simulink library "monroe_library"  (R2012b)
settings: Solver=ode45  StartTime=0.0  StopTime=10.0  RelTol=1e-3
values from neighbouring files (symbols this model uses):
  input_bit_width = ', num2str(input_bit_width))    [fft_direct_draw.m]
undefined symbols (not defined in the file or in its folder): gcbh, xlBlockLoadCallback
libraries: xbsIndex_r4 x1880, monroe_library x159, casper_library x13, xps_library x1
(part 12 of 43)

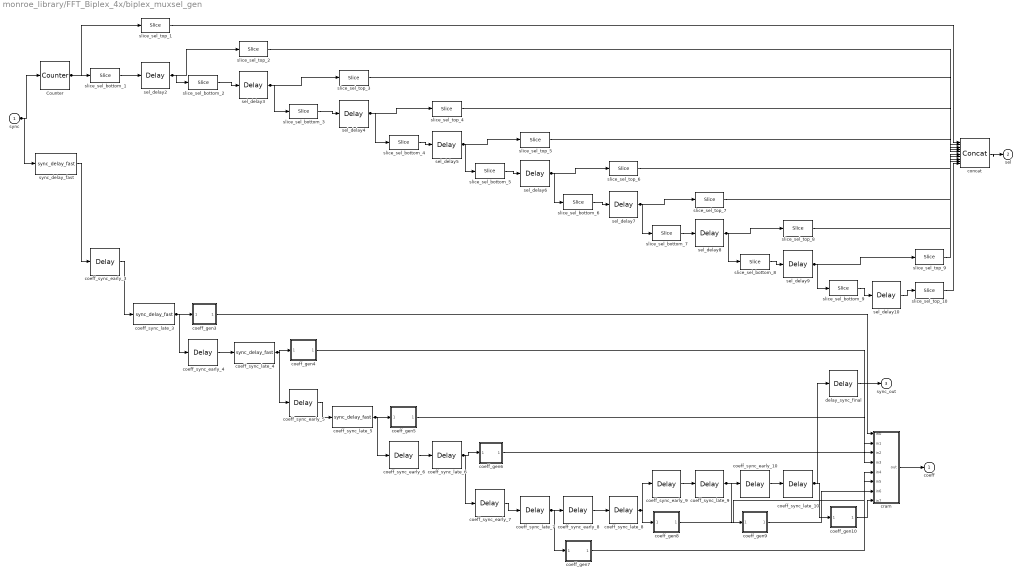
== system monroe_library/FFT_Biplex_4x/biplex_muxsel_gen ==
  sync : Inport
  Counter : xbsIndex_r4/Counter  cnt_type=Free Running  cnt_to=Inf  operation=Up  start_count=0  cnt_by_val=1  arith_type=Unsigned  n_bits=10  bin_pt=0  load_pin=off  rst=on  en=off  explicit_period=on  period=1  dbl_ovrd=off  use_behavioral_HDL=off  implementation=Fabric  block_type=counter
  coeff_gen10 : Subsystem
  coeff_gen3 : Subsystem
  coeff_gen4 : Subsystem
  coeff_gen5 : Subsystem
  coeff_gen6 : Subsystem
  coeff_gen7 : Subsystem
  coeff_gen8 : Subsystem
  coeff_gen9 : Subsystem
  coeff_sync_early_{4..10} (7 alike) : xbsIndex_r4/Delay  en=off  latency=6  dbl_ovrd=off  reg_retiming=off  block_type=delay
  coeff_sync_early_3 : xbsIndex_r4/Delay  en=off  latency=7  dbl_ovrd=off  reg_retiming=off  block_type=delay
  coeff_sync_late_10 : xbsIndex_r4/Delay  en=off  latency=1  dbl_ovrd=off  reg_retiming=off  block_type=delay
  coeff_sync_late_3 : monroe_library/sync_delay_fast  SystemSampleTime=-1  delay_len=128
  coeff_sync_late_4 : monroe_library/sync_delay_fast  SystemSampleTime=-1  delay_len=64
  coeff_sync_late_5 : monroe_library/sync_delay_fast  SystemSampleTime=-1  delay_len=32
  coeff_sync_late_6 : xbsIndex_r4/Delay  en=off  latency=16  dbl_ovrd=off  reg_retiming=off  block_type=delay
  coeff_sync_late_7 : xbsIndex_r4/Delay  en=off  latency=8  dbl_ovrd=off  reg_retiming=off  block_type=delay
  coeff_sync_late_8 : xbsIndex_r4/Delay  en=off  latency=4  dbl_ovrd=off  reg_retiming=off  block_type=delay
  coeff_sync_late_9 : xbsIndex_r4/Delay  en=off  latency=2  dbl_ovrd=off  reg_retiming=off  block_type=delay
  concat : xbsIndex_r4/Concat  num_inputs=10  dbl_ovrd=off  block_type=concat
  cram : Subsystem
  delay_sync_final : xbsIndex_r4/Delay  en=off  latency=6  dbl_ovrd=off  reg_retiming=off  block_type=delay
  sel_delay{4..10} (7 alike) : xbsIndex_r4/Delay  en=off  latency=6  dbl_ovrd=off  reg_retiming=off  block_type=delay
  sel_delay2 : xbsIndex_r4/Delay  en=off  latency=2  dbl_ovrd=off  reg_retiming=off  block_type=delay
  sel_delay3 : xbsIndex_r4/Delay  en=off  latency=5  dbl_ovrd=off  reg_retiming=off  block_type=delay
  slice_sel_bottom_1 : xbsIndex_r4/Slice  nbits=9  boolean_output=off  mode=Lower Bit Location + Width  bit1=0  base1=LSB of Input  bit0=0  base0=LSB of Input  dbl_ovrd=off  block_type=slice
  slice_sel_bottom_2 : xbsIndex_r4/Slice  nbits=8  boolean_output=off  mode=Lower Bit Location + Width  bit1=0  base1=LSB of Input  bit0=0  base0=LSB of Input  dbl_ovrd=off  block_type=slice
  slice_sel_bottom_3 : xbsIndex_r4/Slice  nbits=7  boolean_output=off  mode=Lower Bit Location + Width  bit1=0  base1=LSB of Input  bit0=0  base0=LSB of Input  dbl_ovrd=off  block_type=slice
  slice_sel_bottom_4 : xbsIndex_r4/Slice  nbits=6  boolean_output=off  mode=Lower Bit Location + Width  bit1=0  base1=LSB of Input  bit0=0  base0=LSB of Input  dbl_ovrd=off  block_type=slice
  slice_sel_bottom_5 : xbsIndex_r4/Slice  nbits=5  boolean_output=off  mode=Lower Bit Location + Width  bit1=0  base1=LSB of Input  bit0=0  base0=LSB of Input  dbl_ovrd=off  block_type=slice
  slice_sel_bottom_6 : xbsIndex_r4/Slice  nbits=4  boolean_output=off  mode=Lower Bit Location + Width  bit1=0  base1=LSB of Input  bit0=0  base0=LSB of Input  dbl_ovrd=off  block_type=slice
  slice_sel_bottom_7 : xbsIndex_r4/Slice  nbits=3  boolean_output=off  mode=Lower Bit Location + Width  bit1=0  base1=LSB of Input  bit0=0  base0=LSB of Input  dbl_ovrd=off  block_type=slice
  slice_sel_bottom_8 : xbsIndex_r4/Slice  nbits=2  boolean_output=off  mode=Lower Bit Location + Width  bit1=0  base1=LSB of Input  bit0=0  base0=LSB of Input  dbl_ovrd=off  block_type=slice
  slice_sel_bottom_9 : xbsIndex_r4/Slice  nbits=1  boolean_output=off  mode=Lower Bit Location + Width  bit1=0  base1=LSB of Input  bit0=0  base0=LSB of Input  dbl_ovrd=off  block_type=slice
  slice_sel_top_{1..10} (10 alike) : xbsIndex_r4/Slice  nbits=1  boolean_output=on  mode=Upper Bit Location + Width  bit1=0  base1=MSB of Input  bit0=0  base0=MSB of Input  dbl_ovrd=off  block_type=slice
  sync_delay_fast : monroe_library/sync_delay_fast  SystemSampleTime=-1  delay_len=768
  coeff : Outport
  sel : Outport  Port=2
  sync_out : Outport  Port=3
  wires:
  sync/1 -> Counter/1, sync_delay_fast/1
  coeff_sync_late_3/1 -> coeff_sync_early_4/1, coeff_gen3/1(sync)
  coeff_sync_late_4/1 -> coeff_sync_early_5/1, coeff_gen4/1(sync)
  coeff_sync_late_5/1 -> coeff_sync_early_6/1, coeff_gen5/1(sync)
  coeff_sync_late_6/1 -> coeff_sync_early_7/1, coeff_gen6/1(sync)
  coeff_sync_late_7/1 -> coeff_sync_early_8/1, coeff_gen7/1(sync)
  coeff_sync_late_8/1 -> coeff_sync_early_9/1, coeff_gen8/1(sync)
  coeff_sync_late_9/1 -> coeff_sync_early_10/1, coeff_gen9/1(sync)
  coeff_sync_late_10/1 -> delay_sync_final/1, coeff_gen10/1(sync)
  Counter/1 -> slice_sel_bottom_1/1, slice_sel_top_1/1
  sel_delay2/1 -> slice_sel_bottom_2/1, slice_sel_top_2/1
  sel_delay3/1 -> slice_sel_bottom_3/1, slice_sel_top_3/1
  sel_delay4/1 -> slice_sel_bottom_4/1, slice_sel_top_4/1
  sel_delay5/1 -> slice_sel_bottom_5/1, slice_sel_top_5/1
  sel_delay6/1 -> slice_sel_bottom_6/1, slice_sel_top_6/1
  sel_delay7/1 -> slice_sel_bottom_7/1, slice_sel_top_7/1
  sel_delay8/1 -> slice_sel_bottom_8/1, slice_sel_top_8/1
  sel_delay9/1 -> slice_sel_bottom_9/1, slice_sel_top_9/1
  delay_sync_final/1 -> sync_out/1
  concat/1 -> sel/1
  slice_sel_top_10/1 -> concat/10
  slice_sel_top_9/1 -> concat/9
  slice_sel_top_8/1 -> concat/8
  slice_sel_top_7/1 -> concat/7
  slice_sel_top_6/1 -> concat/6
  slice_sel_top_5/1 -> concat/5
  slice_sel_top_4/1 -> concat/4
  slice_sel_top_3/1 -> concat/3
  slice_sel_top_2/1 -> concat/2
  slice_sel_top_1/1 -> concat/1
  sel_delay10/1 -> slice_sel_top_10/1
  slice_sel_bottom_9/1 -> sel_delay10/1
  slice_sel_bottom_8/1 -> sel_delay9/1
  slice_sel_bottom_7/1 -> sel_delay8/1
  slice_sel_bottom_6/1 -> sel_delay7/1
  slice_sel_bottom_5/1 -> sel_delay6/1
  slice_sel_bottom_4/1 -> sel_delay5/1
  slice_sel_bottom_3/1 -> sel_delay4/1
  slice_sel_bottom_2/1 -> sel_delay3/1
  slice_sel_bottom_1/1 -> sel_delay2/1
  cram/1(out) -> coeff/1
  coeff_gen10/1(coeff) -> cram/8(in7)
  coeff_gen9/1(coeff) -> cram/7(in6)
  coeff_gen8/1(coeff) -> cram/6(in5)
  coeff_gen7/1(coeff) -> cram/5(in4)
  coeff_gen6/1(coeff) -> cram/4(in3)
  coeff_gen5/1(coeff) -> cram/3(in2)
  coeff_gen4/1(coeff) -> cram/2(in1)
  coeff_gen3/1(coeff) -> cram/1(in0)
  coeff_sync_early_10/1 -> coeff_sync_late_10/1
  coeff_sync_early_9/1 -> coeff_sync_late_9/1
  coeff_sync_early_8/1 -> coeff_sync_late_8/1
  coeff_sync_early_7/1 -> coeff_sync_late_7/1
  coeff_sync_early_6/1 -> coeff_sync_late_6/1
  coeff_sync_early_5/1 -> coeff_sync_late_5/1
  coeff_sync_early_4/1 -> coeff_sync_late_4/1
  coeff_sync_early_3/1 -> coeff_sync_late_3/1
  sync_delay_fast/1 -> coeff_sync_early_3/1

== system monroe_library/FFT_Biplex_4x/cram0 ==
  in0 : Inport
  in1 : Inport  Port=2
  concat : xbsIndex_r4/Concat  num_inputs=2  dbl_ovrd=off  block_type=concat
  reinterpret_1 : xbsIndex_r4/Reinterpret  force_arith_type=on  arith_type=Unsigned  force_bin_pt=on  bin_pt=0  block_type=reinterpret
      settings: infoedit="Changes signal type without altering the binary representation.   You can changed the signal between signed and unsigned, and relocate the binary point.<br><br>Hardware notes: In hardware this block costs nothing.<br><br>Example:  Suppose the input is 6 bits wide, signed, with 2 fractional bits, and the output is forced to unsigned with 0 fractional bits.  Then an input of -2.0 (1110.00 in binary 2's complement) becomes an output of 56 (111000 in binary)."
  reinterpret_2 : xbsIndex_r4/Reinterpret  force_arith_type=on  arith_type=Unsigned  force_bin_pt=on  bin_pt=0  block_type=reinterpret
      settings: infoedit="Changes signal type without altering the binary representation.   You can changed the signal between signed and unsigned, and relocate the binary point.<br><br>Hardware notes: In hardware this block costs nothing.<br><br>Example:  Suppose the input is 6 bits wide, signed, with 2 fractional bits, and the output is forced to unsigned with 0 fractional bits.  Then an input of -2.0 (1110.00 in binary 2's complement) becomes an output of 56 (111000 in binary)."
  out : Outport
  wires:
  concat/1 -> out/1
  reinterpret_2/1 -> concat/2
  reinterpret_1/1 -> concat/1
  in1/1 -> reinterpret_2/1
  in0/1 -> reinterpret_1/1

== system monroe_library/FFT_Biplex_4x/cram1 ==
  in0 : Inport
  in1 : Inport  Port=2
  concat : xbsIndex_r4/Concat  num_inputs=2  dbl_ovrd=off  block_type=concat
  reinterpret_1 : xbsIndex_r4/Reinterpret  force_arith_type=on  arith_type=Unsigned  force_bin_pt=on  bin_pt=0  block_type=reinterpret
      settings: infoedit="Changes signal type without altering the binary representation.   You can changed the signal between signed and unsigned, and relocate the binary point.<br><br>Hardware notes: In hardware this block costs nothing.<br><br>Example:  Suppose the input is 6 bits wide, signed, with 2 fractional bits, and the output is forced to unsigned with 0 fractional bits.  Then an input of -2.0 (1110.00 in binary 2's complement) becomes an output of 56 (111000 in binary)."
  reinterpret_2 : xbsIndex_r4/Reinterpret  force_arith_type=on  arith_type=Unsigned  force_bin_pt=on  bin_pt=0  block_type=reinterpret
      settings: infoedit="Changes signal type without altering the binary representation.   You can changed the signal between signed and unsigned, and relocate the binary point.<br><br>Hardware notes: In hardware this block costs nothing.<br><br>Example:  Suppose the input is 6 bits wide, signed, with 2 fractional bits, and the output is forced to unsigned with 0 fractional bits.  Then an input of -2.0 (1110.00 in binary 2's complement) becomes an output of 56 (111000 in binary)."
  out : Outport
  wires:
  concat/1 -> out/1
  reinterpret_2/1 -> concat/2
  reinterpret_1/1 -> concat/1
  in1/1 -> reinterpret_2/1
  in0/1 -> reinterpret_1/1

== system monroe_library/FFT_Biplex_4x/stage_1 ==
  a : Inport
  b : Inport  Port=2
  sync : Inport  Port=3
  mux_sel : Inport  Port=4
  Mux : xbsIndex_r4/Mux  inputs=2  en=off  latency=0  precision=Full  arith_type="Signed  (2's comp)"  n_bits=8  bin_pt=2  quantization=Truncate  overflow=Wrap  dbl_ovrd=off  block_type=mux
  Mux1 : xbsIndex_r4/Mux  inputs=2  en=off  latency=0  precision=Full  arith_type="Signed  (2's comp)"  n_bits=8  bin_pt=2  quantization=Truncate  overflow=Wrap  dbl_ovrd=off  block_type=mux
  double_delay_bram_fast : monroe_library/double_delay_bram_fast  SystemSampleTime=-1  delay_len=512  bram_latency=2  register_counter=0
  sync_delay_fast1 : monroe_library/sync_delay_fast  SystemSampleTime=-1  delay_len=512
  twiddle_stage1 : monroe_library/twiddle_stage1  SystemSampleTime=-1  input_bit_width=18  out_n_bits=18  downshift_at_end=1
  a+bw : Outport
  a-bw : Outport  Port=2
  sync_out : Outport  Port=3
  wires:
  mux_sel/1 -> Mux1/1, Mux/1
  double_delay_bram_fast/2 -> Mux1/3, Mux/2
  a/1 -> Mux1/2, Mux/3
  twiddle_stage1/3 -> sync_out/1
  twiddle_stage1/2 -> a-bw/1
  twiddle_stage1/1 -> a+bw/1
  sync_delay_fast1/1 -> twiddle_stage1/3
  Mux/1 -> twiddle_stage1/2
  double_delay_bram_fast/1 -> twiddle_stage1/1
  sync/1 -> sync_delay_fast1/1
  b/1 -> double_delay_bram_fast/2
  Mux1/1 -> double_delay_bram_fast/1

== system monroe_library/FFT_Biplex_4x/stage_10 ==
  a : Inport
  b : Inport  Port=2
  sync : Inport  Port=3
  coeff : Inport  Port=4
  mux_sel : Inport  Port=5
  Mux : xbsIndex_r4/Mux  inputs=2  en=off  latency=0  precision=Full  arith_type="Signed  (2's comp)"  n_bits=8  bin_pt=2  quantization=Truncate  overflow=Wrap  dbl_ovrd=off  block_type=mux
  Mux1 : xbsIndex_r4/Mux  inputs=2  en=off  latency=0  precision=Full  arith_type="Signed  (2's comp)"  n_bits=8  bin_pt=2  quantization=Truncate  overflow=Wrap  dbl_ovrd=off  block_type=mux
  delay_ddbf_1 : xbsIndex_r4/Delay  en=off  latency=1  dbl_ovrd=off  reg_retiming=off  block_type=delay
  delay_ddbf_2 : xbsIndex_r4/Delay  en=off  latency=1  dbl_ovrd=off  reg_retiming=off  block_type=delay
  delay_end : xbsIndex_r4/Delay  en=off  latency=2  dbl_ovrd=off  reg_retiming=off  block_type=delay
  delay_mid : xbsIndex_r4/Delay  en=off  latency=1  dbl_ovrd=off  reg_retiming=off  block_type=delay
  sync_delay : xbsIndex_r4/Delay  en=off  latency=1  dbl_ovrd=off  reg_retiming=off  block_type=delay
  twiddle_cheap : monroe_library/twiddle_cheap  SystemSampleTime=-1  a_n_bits=18  a_bin_pt=17  b_n_bits=18  b_bin_pt=17  w_n_bits=18  w_bin_pt=17  a_delay=0  apbw_delay=0  out_n_bits=18  downshift_at_end=1
  a+bw : Outport
  a-bw : Outport  Port=2
  sync_out : Outport  Port=3
  wires:
  mux_sel/1 -> Mux1/1, Mux/1
  delay_ddbf_2/1 -> Mux1/3, Mux/2
  a/1 -> Mux1/2, Mux/3
  twiddle_cheap/3 -> sync_out/1
  twiddle_cheap/2 -> a-bw/1
  twiddle_cheap/1 -> delay_end/1
  sync_delay/1 -> twiddle_cheap/4
  coeff/1 -> twiddle_cheap/3
  Mux/1 -> twiddle_cheap/2
  delay_mid/1 -> twiddle_cheap/1
  sync/1 -> sync_delay/1
  b/1 -> delay_ddbf_2/1
  delay_ddbf_1/1 -> delay_mid/1
  delay_end/1 -> a+bw/1
  Mux1/1 -> delay_ddbf_1/1

== system monroe_library/FFT_Biplex_4x/stage_2 ==
  a : Inport
  b : Inport  Port=2
  sync : Inport  Port=3
  mux_sel : Inport  Port=4
  Mux : xbsIndex_r4/Mux  inputs=2  en=off  latency=0  precision=Full  arith_type="Signed  (2's comp)"  n_bits=8  bin_pt=2  quantization=Truncate  overflow=Wrap  dbl_ovrd=off  block_type=mux
  Mux1 : xbsIndex_r4/Mux  inputs=2  en=off  latency=0  precision=Full  arith_type="Signed  (2's comp)"  n_bits=8  bin_pt=2  quantization=Truncate  overflow=Wrap  dbl_ovrd=off  block_type=mux
  double_delay_bram_fast : monroe_library/double_delay_bram_fast  SystemSampleTime=-1  delay_len=256  bram_latency=2  register_counter=0
  sync_delay_fast2 : monroe_library/sync_delay_fast  SystemSampleTime=-1  delay_len=256
  twiddle_stage2 : monroe_library/twiddle_stage2  SystemSampleTime=-1  FFTSize=10  input_bit_width=18  out_n_bits=18  downshift_at_end=1
  a+bw : Outport
  a-bw : Outport  Port=2
  sync_out : Outport  Port=3
  wires:
  mux_sel/1 -> twiddle_stage2/3, Mux1/1, Mux/1
  double_delay_bram_fast/2 -> Mux1/3, Mux/2
  a/1 -> Mux1/2, Mux/3
  twiddle_stage2/3 -> sync_out/1
  twiddle_stage2/2 -> a-bw/1
  twiddle_stage2/1 -> a+bw/1
  sync_delay_fast2/1 -> twiddle_stage2/4
  Mux/1 -> twiddle_stage2/2
  double_delay_bram_fast/1 -> twiddle_stage2/1
  sync/1 -> sync_delay_fast2/1
  b/1 -> double_delay_bram_fast/2
  Mux1/1 -> double_delay_bram_fast/1

== system monroe_library/FFT_Biplex_4x/stage_3 ==
  a : Inport
  b : Inport  Port=2
  sync : Inport  Port=3
  coeff : Inport  Port=4
  mux_sel : Inport  Port=5
  Mux : xbsIndex_r4/Mux  inputs=2  en=off  latency=0  precision=Full  arith_type="Signed  (2's comp)"  n_bits=8  bin_pt=2  quantization=Truncate  overflow=Wrap  dbl_ovrd=off  block_type=mux
  Mux1 : xbsIndex_r4/Mux  inputs=2  en=off  latency=0  precision=Full  arith_type="Signed  (2's comp)"  n_bits=8  bin_pt=2  quantization=Truncate  overflow=Wrap  dbl_ovrd=off  block_type=mux
  delay_end : xbsIndex_r4/Delay  en=off  latency=2  dbl_ovrd=off  reg_retiming=off  block_type=delay
  delay_mid : xbsIndex_r4/Delay  en=off  latency=1  dbl_ovrd=off  reg_retiming=off  block_type=delay
  double_delay_bram_fast : monroe_library/double_delay_bram_fast  SystemSampleTime=-1  delay_len=128  bram_latency=2  register_counter=0
  sync_delay_fast3 : monroe_library/sync_delay_fast  SystemSampleTime=-1  delay_len=128
  twiddle_cheap : monroe_library/twiddle_cheap  SystemSampleTime=-1  a_n_bits=18  a_bin_pt=17  b_n_bits=18  b_bin_pt=17  w_n_bits=18  w_bin_pt=17  a_delay=0  apbw_delay=0  out_n_bits=18  downshift_at_end=1
  a+bw : Outport
  a-bw : Outport  Port=2
  sync_out : Outport  Port=3
  wires:
  mux_sel/1 -> Mux1/1, Mux/1
  double_delay_bram_fast/2 -> Mux1/3, Mux/2
  a/1 -> Mux1/2, Mux/3
  twiddle_cheap/3 -> sync_out/1
  twiddle_cheap/2 -> a-bw/1
  twiddle_cheap/1 -> delay_end/1
  sync_delay_fast3/1 -> twiddle_cheap/4
  coeff/1 -> twiddle_cheap/3
  Mux/1 -> twiddle_cheap/2
  delay_mid/1 -> twiddle_cheap/1
  sync/1 -> sync_delay_fast3/1
  b/1 -> double_delay_bram_fast/2
  double_delay_bram_fast/1 -> delay_mid/1
  delay_end/1 -> a+bw/1
  Mux1/1 -> double_delay_bram_fast/1

== system monroe_library/FFT_Biplex_4x/stage_4 ==
  a : Inport
  b : Inport  Port=2
  sync : Inport  Port=3
  coeff : Inport  Port=4
  mux_sel : Inport  Port=5
  Mux : xbsIndex_r4/Mux  inputs=2  en=off  latency=0  precision=Full  arith_type="Signed  (2's comp)"  n_bits=8  bin_pt=2  quantization=Truncate  overflow=Wrap  dbl_ovrd=off  block_type=mux
  Mux1 : xbsIndex_r4/Mux  inputs=2  en=off  latency=0  precision=Full  arith_type="Signed  (2's comp)"  n_bits=8  bin_pt=2  quantization=Truncate  overflow=Wrap  dbl_ovrd=off  block_type=mux
  delay_end : xbsIndex_r4/Delay  en=off  latency=2  dbl_ovrd=off  reg_retiming=off  block_type=delay
  delay_mid : xbsIndex_r4/Delay  en=off  latency=1  dbl_ovrd=off  reg_retiming=off  block_type=delay
  double_delay_bram_fast : monroe_library/double_delay_bram_fast  SystemSampleTime=-1  delay_len=64  bram_latency=2  register_counter=0
  sync_delay_fast4 : monroe_library/sync_delay_fast  SystemSampleTime=-1  delay_len=64
  twiddle_cheap : monroe_library/twiddle_cheap  SystemSampleTime=-1  a_n_bits=18  a_bin_pt=17  b_n_bits=18  b_bin_pt=17  w_n_bits=18  w_bin_pt=17  a_delay=0  apbw_delay=0  out_n_bits=18  downshift_at_end=1
  a+bw : Outport
  a-bw : Outport  Port=2
  sync_out : Outport  Port=3
  wires:
  mux_sel/1 -> Mux1/1, Mux/1
  double_delay_bram_fast/2 -> Mux1/3, Mux/2
  a/1 -> Mux1/2, Mux/3
  twiddle_cheap/3 -> sync_out/1
  twiddle_cheap/2 -> a-bw/1
  twiddle_cheap/1 -> delay_end/1
  sync_delay_fast4/1 -> twiddle_cheap/4
  coeff/1 -> twiddle_cheap/3
  Mux/1 -> twiddle_cheap/2
  delay_mid/1 -> twiddle_cheap/1
  sync/1 -> sync_delay_fast4/1
  b/1 -> double_delay_bram_fast/2
  double_delay_bram_fast/1 -> delay_mid/1
  delay_end/1 -> a+bw/1
  Mux1/1 -> double_delay_bram_fast/1

== system monroe_library/FFT_Biplex_4x/stage_5 ==
  a : Inport
  b : Inport  Port=2
  sync : Inport  Port=3
  coeff : Inport  Port=4
  mux_sel : Inport  Port=5
  Mux : xbsIndex_r4/Mux  inputs=2  en=off  latency=0  precision=Full  arith_type="Signed  (2's comp)"  n_bits=8  bin_pt=2  quantization=Truncate  overflow=Wrap  dbl_ovrd=off  block_type=mux
  Mux1 : xbsIndex_r4/Mux  inputs=2  en=off  latency=0  precision=Full  arith_type="Signed  (2's comp)"  n_bits=8  bin_pt=2  quantization=Truncate  overflow=Wrap  dbl_ovrd=off  block_type=mux
  delay_end : xbsIndex_r4/Delay  en=off  latency=2  dbl_ovrd=off  reg_retiming=off  block_type=delay
  delay_mid : xbsIndex_r4/Delay  en=off  latency=1  dbl_ovrd=off  reg_retiming=off  block_type=delay
  double_delay_bram_fast : monroe_library/double_delay_bram_fast  SystemSampleTime=-1  delay_len=32  bram_latency=2  register_counter=0
  sync_delay_fast5 : monroe_library/sync_delay_fast  SystemSampleTime=-1  delay_len=32
  twiddle_cheap : monroe_library/twiddle_cheap  SystemSampleTime=-1  a_n_bits=18  a_bin_pt=17  b_n_bits=18  b_bin_pt=17  w_n_bits=18  w_bin_pt=17  a_delay=0  apbw_delay=0  out_n_bits=18  downshift_at_end=1
  a+bw : Outport
  a-bw : Outport  Port=2
  sync_out : Outport  Port=3
  wires:
  mux_sel/1 -> Mux1/1, Mux/1
  double_delay_bram_fast/2 -> Mux1/3, Mux/2
  a/1 -> Mux1/2, Mux/3
  twiddle_cheap/3 -> sync_out/1
  twiddle_cheap/2 -> a-bw/1
  twiddle_cheap/1 -> delay_end/1
  sync_delay_fast5/1 -> twiddle_cheap/4
  coeff/1 -> twiddle_cheap/3
  Mux/1 -> twiddle_cheap/2
  delay_mid/1 -> twiddle_cheap/1
  sync/1 -> sync_delay_fast5/1
  b/1 -> double_delay_bram_fast/2
  double_delay_bram_fast/1 -> delay_mid/1
  delay_end/1 -> a+bw/1
  Mux1/1 -> double_delay_bram_fast/1

== system monroe_library/FFT_Biplex_4x/stage_6 ==
  a : Inport
  b : Inport  Port=2
  sync : Inport  Port=3
  coeff : Inport  Port=4
  mux_sel : Inport  Port=5
  Mux : xbsIndex_r4/Mux  inputs=2  en=off  latency=0  precision=Full  arith_type="Signed  (2's comp)"  n_bits=8  bin_pt=2  quantization=Truncate  overflow=Wrap  dbl_ovrd=off  block_type=mux
  Mux1 : xbsIndex_r4/Mux  inputs=2  en=off  latency=0  precision=Full  arith_type="Signed  (2's comp)"  n_bits=8  bin_pt=2  quantization=Truncate  overflow=Wrap  dbl_ovrd=off  block_type=mux
  delay_end : xbsIndex_r4/Delay  en=off  latency=2  dbl_ovrd=off  reg_retiming=off  block_type=delay
  delay_mid : xbsIndex_r4/Delay  en=off  latency=1  dbl_ovrd=off  reg_retiming=off  block_type=delay
  double_delay_bram_fast : monroe_library/double_delay_bram_fast  SystemSampleTime=-1  delay_len=16  bram_latency=2  register_counter=0
  sync_delay : xbsIndex_r4/Delay  en=off  latency=16  dbl_ovrd=off  reg_retiming=off  block_type=delay
  twiddle_cheap : monroe_library/twiddle_cheap  SystemSampleTime=-1  a_n_bits=18  a_bin_pt=17  b_n_bits=18  b_bin_pt=17  w_n_bits=18  w_bin_pt=17  a_delay=0  apbw_delay=0  out_n_bits=18  downshift_at_end=1
  a+bw : Outport
  a-bw : Outport  Port=2
  sync_out : Outport  Port=3
  wires:
  mux_sel/1 -> Mux1/1, Mux/1
  double_delay_bram_fast/2 -> Mux1/3, Mux/2
  a/1 -> Mux1/2, Mux/3
  twiddle_cheap/3 -> sync_out/1
  twiddle_cheap/2 -> a-bw/1
  twiddle_cheap/1 -> delay_end/1
  sync_delay/1 -> twiddle_cheap/4
  coeff/1 -> twiddle_cheap/3
  Mux/1 -> twiddle_cheap/2
  delay_mid/1 -> twiddle_cheap/1
  sync/1 -> sync_delay/1
  b/1 -> double_delay_bram_fast/2
  double_delay_bram_fast/1 -> delay_mid/1
  delay_end/1 -> a+bw/1
  Mux1/1 -> double_delay_bram_fast/1

== system monroe_library/FFT_Biplex_4x/stage_7 ==
  a : Inport
  b : Inport  Port=2
  sync : Inport  Port=3
  coeff : Inport  Port=4
  mux_sel : Inport  Port=5
  Mux : xbsIndex_r4/Mux  inputs=2  en=off  latency=0  precision=Full  arith_type="Signed  (2's comp)"  n_bits=8  bin_pt=2  quantization=Truncate  overflow=Wrap  dbl_ovrd=off  block_type=mux
  Mux1 : xbsIndex_r4/Mux  inputs=2  en=off  latency=0  precision=Full  arith_type="Signed  (2's comp)"  n_bits=8  bin_pt=2  quantization=Truncate  overflow=Wrap  dbl_ovrd=off  block_type=mux
  delay_ddbf_1 : xbsIndex_r4/Delay  en=off  latency=8  dbl_ovrd=off  reg_retiming=off  block_type=delay
  delay_ddbf_2 : xbsIndex_r4/Delay  en=off  latency=8  dbl_ovrd=off  reg_retiming=off  block_type=delay
  delay_end : xbsIndex_r4/Delay  en=off  latency=2  dbl_ovrd=off  reg_retiming=off  block_type=delay
  delay_mid : xbsIndex_r4/Delay  en=off  latency=1  dbl_ovrd=off  reg_retiming=off  block_type=delay
  sync_delay : xbsIndex_r4/Delay  en=off  latency=8  dbl_ovrd=off  reg_retiming=off  block_type=delay
  twiddle_cheap : monroe_library/twiddle_cheap  SystemSampleTime=-1  a_n_bits=18  a_bin_pt=17  b_n_bits=18  b_bin_pt=17  w_n_bits=18  w_bin_pt=17  a_delay=0  apbw_delay=0  out_n_bits=18  downshift_at_end=1
  a+bw : Outport
  a-bw : Outport  Port=2
  sync_out : Outport  Port=3
  wires:
  mux_sel/1 -> Mux1/1, Mux/1
  delay_ddbf_2/1 -> Mux1/3, Mux/2
  a/1 -> Mux1/2, Mux/3
  twiddle_cheap/3 -> sync_out/1
  twiddle_cheap/2 -> a-bw/1
  twiddle_cheap/1 -> delay_end/1
  sync_delay/1 -> twiddle_cheap/4
  coeff/1 -> twiddle_cheap/3
  Mux/1 -> twiddle_cheap/2
  delay_mid/1 -> twiddle_cheap/1
  sync/1 -> sync_delay/1
  b/1 -> delay_ddbf_2/1
  delay_ddbf_1/1 -> delay_mid/1
  delay_end/1 -> a+bw/1
  Mux1/1 -> delay_ddbf_1/1

== system monroe_library/FFT_Biplex_4x/stage_8 ==
  a : Inport
  b : Inport  Port=2
  sync : Inport  Port=3
  coeff : Inport  Port=4
  mux_sel : Inport  Port=5
  Mux : xbsIndex_r4/Mux  inputs=2  en=off  latency=0  precision=Full  arith_type="Signed  (2's comp)"  n_bits=8  bin_pt=2  quantization=Truncate  overflow=Wrap  dbl_ovrd=off  block_type=mux
  Mux1 : xbsIndex_r4/Mux  inputs=2  en=off  latency=0  precision=Full  arith_type="Signed  (2's comp)"  n_bits=8  bin_pt=2  quantization=Truncate  overflow=Wrap  dbl_ovrd=off  block_type=mux
  delay_ddbf_1 : xbsIndex_r4/Delay  en=off  latency=4  dbl_ovrd=off  reg_retiming=off  block_type=delay
  delay_ddbf_2 : xbsIndex_r4/Delay  en=off  latency=4  dbl_ovrd=off  reg_retiming=off  block_type=delay
  delay_end : xbsIndex_r4/Delay  en=off  latency=2  dbl_ovrd=off  reg_retiming=off  block_type=delay
  delay_mid : xbsIndex_r4/Delay  en=off  latency=1  dbl_ovrd=off  reg_retiming=off  block_type=delay
  sync_delay : xbsIndex_r4/Delay  en=off  latency=4  dbl_ovrd=off  reg_retiming=off  block_type=delay
  twiddle_cheap : monroe_library/twiddle_cheap  SystemSampleTime=-1  a_n_bits=18  a_bin_pt=17  b_n_bits=18  b_bin_pt=17  w_n_bits=18  w_bin_pt=17  a_delay=0  apbw_delay=0  out_n_bits=18  downshift_at_end=1
  a+bw : Outport
  a-bw : Outport  Port=2
  sync_out : Outport  Port=3
  wires:
  mux_sel/1 -> Mux1/1, Mux/1
  delay_ddbf_2/1 -> Mux1/3, Mux/2
  a/1 -> Mux1/2, Mux/3
  twiddle_cheap/3 -> sync_out/1
  twiddle_cheap/2 -> a-bw/1
  twiddle_cheap/1 -> delay_end/1
  sync_delay/1 -> twiddle_cheap/4
  coeff/1 -> twiddle_cheap/3
  Mux/1 -> twiddle_cheap/2
  delay_mid/1 -> twiddle_cheap/1
  sync/1 -> sync_delay/1
  b/1 -> delay_ddbf_2/1
  delay_ddbf_1/1 -> delay_mid/1
  delay_end/1 -> a+bw/1
  Mux1/1 -> delay_ddbf_1/1

== system monroe_library/FFT_Biplex_4x/stage_9 ==
  a : Inport
  b : Inport  Port=2
  sync : Inport  Port=3
  coeff : Inport  Port=4
  mux_sel : Inport  Port=5
  Mux : xbsIndex_r4/Mux  inputs=2  en=off  latency=0  precision=Full  arith_type="Signed  (2's comp)"  n_bits=8  bin_pt=2  quantization=Truncate  overflow=Wrap  dbl_ovrd=off  block_type=mux
  Mux1 : xbsIndex_r4/Mux  inputs=2  en=off  latency=0  precision=Full  arith_type="Signed  (2's comp)"  n_bits=8  bin_pt=2  quantization=Truncate  overflow=Wrap  dbl_ovrd=off  block_type=mux
  delay_ddbf_1 : xbsIndex_r4/Delay  en=off  latency=2  dbl_ovrd=off  reg_retiming=off  block_type=delay
  delay_ddbf_2 : xbsIndex_r4/Delay  en=off  latency=2  dbl_ovrd=off  reg_retiming=off  block_type=delay
  delay_end : xbsIndex_r4/Delay  en=off  latency=2  dbl_ovrd=off  reg_retiming=off  block_type=delay
  delay_mid : xbsIndex_r4/Delay  en=off  latency=1  dbl_ovrd=off  reg_retiming=off  block_type=delay
  sync_delay : xbsIndex_r4/Delay  en=off  latency=2  dbl_ovrd=off  reg_retiming=off  block_type=delay
  twiddle_cheap : monroe_library/twiddle_cheap  SystemSampleTime=-1  a_n_bits=18  a_bin_pt=17  b_n_bits=18  b_bin_pt=17  w_n_bits=18  w_bin_pt=17  a_delay=0  apbw_delay=0  out_n_bits=18  downshift_at_end=1
  a+bw : Outport
  a-bw : Outport  Port=2
  sync_out : Outport  Port=3
  wires:
  mux_sel/1 -> Mux1/1, Mux/1
  delay_ddbf_2/1 -> Mux1/3, Mux/2
  a/1 -> Mux1/2, Mux/3
  twiddle_cheap/3 -> sync_out/1
  twiddle_cheap/2 -> a-bw/1
  twiddle_cheap/1 -> delay_end/1
  sync_delay/1 -> twiddle_cheap/4
  coeff/1 -> twiddle_cheap/3
  Mux/1 -> twiddle_cheap/2
  delay_mid/1 -> twiddle_cheap/1
  sync/1 -> sync_delay/1
  b/1 -> delay_ddbf_2/1
  delay_ddbf_1/1 -> delay_mid/1
  delay_end/1 -> a+bw/1
  Mux1/1 -> delay_ddbf_1/1

== system monroe_library/FFT_direct/bulk_delay_0_1 ==
  in1 : Inport
  in2 : Inport  Port=2
  in3 : Inport  Port=3
  in4 : Inport  Port=4
  in5 : Inport  Port=5
  in6 : Inport  Port=6
  in7 : Inport  Port=7
  in8 : Inport  Port=8
  delay_{1,3,5,7} (4 alike) : xbsIndex_r4/Delay  en=off  latency=2  dbl_ovrd=off  reg_retiming=off  block_type=delay
  delay_{2,4,6,8} (4 alike) : xbsIndex_r4/Delay  en=off  latency=1  dbl_ovrd=off  reg_retiming=off  block_type=delay
  out1 : Outport
  out2 : Outport  Port=2
  out3 : Outport  Port=3
  out4 : Outport  Port=4
  out5 : Outport  Port=5
  out6 : Outport  Port=6
  out7 : Outport  Port=7
  out8 : Outport  Port=8
  wires:
  delay_8/1 -> out8/1
  in8/1 -> delay_8/1
  delay_7/1 -> out7/1
  in7/1 -> delay_7/1
  delay_6/1 -> out6/1
  in6/1 -> delay_6/1
  delay_5/1 -> out5/1
  in5/1 -> delay_5/1
  delay_4/1 -> out4/1
  in4/1 -> delay_4/1
  delay_3/1 -> out3/1
  in3/1 -> delay_3/1
  delay_2/1 -> out2/1
  in2/1 -> delay_2/1
  delay_1/1 -> out1/1
  in1/1 -> delay_1/1

== system monroe_library/FFT_direct/bulk_delay_1_1 ==
  in1 : Inport
  in2 : Inport  Port=2
  in3 : Inport  Port=3
  in4 : Inport  Port=4
  in5 : Inport  Port=5
  in6 : Inport  Port=6
  in7 : Inport  Port=7
  in8 : Inport  Port=8
  delay_1 : xbsIndex_r4/Delay  en=off  latency=4  dbl_ovrd=off  reg_retiming=off  block_type=delay
  delay_2 : xbsIndex_r4/Delay  en=off  latency=3  dbl_ovrd=off  reg_retiming=off  block_type=delay
  delay_3 : xbsIndex_r4/Delay  en=off  latency=4  dbl_ovrd=off  reg_retiming=off  block_type=delay
  delay_4 : xbsIndex_r4/Delay  en=off  latency=3  dbl_ovrd=off  reg_retiming=off  block_type=delay
  delay_5 : xbsIndex_r4/Delay  en=off  latency=2  dbl_ovrd=off  reg_retiming=off  block_type=delay
  delay_6 : xbsIndex_r4/Delay  en=off  latency=1  dbl_ovrd=off  reg_retiming=off  block_type=delay
  delay_7 : xbsIndex_r4/Delay  en=off  latency=2  dbl_ovrd=off  reg_retiming=off  block_type=delay
  delay_8 : xbsIndex_r4/Delay  en=off  latency=1  dbl_ovrd=off  reg_retiming=off  block_type=delay
  out1 : Outport
  out2 : Outport  Port=2
  out3 : Outport  Port=3
  out4 : Outport  Port=4
  out5 : Outport  Port=5
  out6 : Outport  Port=6
  out7 : Outport  Port=7
  out8 : Outport  Port=8
  wires:
  delay_8/1 -> out8/1
  in8/1 -> delay_8/1
  delay_7/1 -> out7/1
  in7/1 -> delay_7/1
  delay_6/1 -> out6/1
  in6/1 -> delay_6/1
  delay_5/1 -> out5/1
  in5/1 -> delay_5/1
  delay_4/1 -> out4/1
  in4/1 -> delay_4/1
  delay_3/1 -> out3/1
  in3/1 -> delay_3/1
  delay_2/1 -> out2/1
  in2/1 -> delay_2/1
  delay_1/1 -> out1/1
  in1/1 -> delay_1/1

== system monroe_library/FFT_direct/bulk_delay_2_1 ==
  in1 : Inport
  in2 : Inport  Port=2
  in3 : Inport  Port=3
  in4 : Inport  Port=4
  in5 : Inport  Port=5
  in6 : Inport  Port=6
  in7 : Inport  Port=7
  in8 : Inport  Port=8
  delay_1 : xbsIndex_r4/Delay  en=off  latency=4  dbl_ovrd=off  reg_retiming=off  block_type=delay
  delay_2 : xbsIndex_r4/Delay  en=off  latency=3  dbl_ovrd=off  reg_retiming=off  block_type=delay
  delay_3 : xbsIndex_r4/Delay  en=off  latency=2  dbl_ovrd=off  reg_retiming=off  block_type=delay
  delay_4 : xbsIndex_r4/Delay  en=off  latency=1  dbl_ovrd=off  reg_retiming=off  block_type=delay
  delay_5 : xbsIndex_r4/Delay  en=off  latency=4  dbl_ovrd=off  reg_retiming=off  block_type=delay
  delay_6 : xbsIndex_r4/Delay  en=off  latency=3  dbl_ovrd=off  reg_retiming=off  block_type=delay
  delay_7 : xbsIndex_r4/Delay  en=off  latency=2  dbl_ovrd=off  reg_retiming=off  block_type=delay
  delay_8 : xbsIndex_r4/Delay  en=off  latency=1  dbl_ovrd=off  reg_retiming=off  block_type=delay
  out1 : Outport
  out2 : Outport  Port=2
  out3 : Outport  Port=3
  out4 : Outport  Port=4
  out5 : Outport  Port=5
  out6 : Outport  Port=6
  out7 : Outport  Port=7
  out8 : Outport  Port=8
  wires:
  delay_8/1 -> out8/1
  in8/1 -> delay_8/1
  delay_7/1 -> out7/1
  in7/1 -> delay_7/1
  delay_6/1 -> out6/1
  in6/1 -> delay_6/1
  delay_5/1 -> out5/1
  in5/1 -> delay_5/1
  delay_4/1 -> out4/1
  in4/1 -> delay_4/1
  delay_3/1 -> out3/1
  in3/1 -> delay_3/1
  delay_2/1 -> out2/1
  in2/1 -> delay_2/1
  delay_1/1 -> out1/1
  in1/1 -> delay_1/1

== system monroe_library/FFT_direct/bulk_delay_3_1 ==
  in1 : Inport
  in2 : Inport  Port=2
  in3 : Inport  Port=3
  in4 : Inport  Port=4
  in5 : Inport  Port=5
  in6 : Inport  Port=6
  in7 : Inport  Port=7
  in8 : Inport  Port=8
  delay_{1..4} (4 alike) : xbsIndex_r4/Delay  en=off  latency=2  dbl_ovrd=off  reg_retiming=off  block_type=delay
  out1 : Outport
  out2 : Outport  Port=2
  out3 : Outport  Port=3
  out4 : Outport  Port=4
  out5 : Outport  Port=5
  out6 : Outport  Port=6
  out7 : Outport  Port=7
  out8 : Outport  Port=8
  wires:
  in8/1 -> out8/1
  in7/1 -> out7/1
  in6/1 -> out6/1
  in5/1 -> out5/1
  delay_4/1 -> out4/1
  in4/1 -> delay_4/1
  delay_3/1 -> out3/1
  in3/1 -> delay_3/1
  delay_2/1 -> out2/1
  in2/1 -> delay_2/1
  delay_1/1 -> out1/1
  in1/1 -> delay_1/1

== system monroe_library/FFT_direct/direct_coeff_gen ==
  sync : Inport
  bulk_delay_1_1 : Subsystem
  bulk_delay_1_2 : Subsystem
  bulk_delay_2_1 : Subsystem
  bulk_delay_2_2 : Subsystem
  bulk_delay_3_1 : Subsystem
  bulk_delay_3_2 : Subsystem
  coeff_gen_stage_1_group_1 : Subsystem
  coeff_gen_stage_1_group_2 : Subsystem
  coeff_gen_stage_1_group_3 : Subsystem
  coeff_gen_stage_1_group_4 : Subsystem
  coeff_gen_stage_2_group_1 : Subsystem
  coeff_gen_stage_2_group_2 : Subsystem
  coeff_gen_stage_2_group_3 : Subsystem
  coeff_gen_stage_2_group_4 : Subsystem
  coeff_gen_stage_3_group_1 : Subsystem
  coeff_gen_stage_3_group_2 : Subsystem
  coeff_gen_stage_3_group_3 : Subsystem
  coeff_gen_stage_3_group_4 : Subsystem
  concat_stage_1 : xbsIndex_r4/Concat  num_inputs=4  dbl_ovrd=off  block_type=concat
  concat_stage_2 : xbsIndex_r4/Concat  num_inputs=4  dbl_ovrd=off  block_type=concat
  concat_stage_3 : xbsIndex_r4/Concat  num_inputs=4  dbl_ovrd=off  block_type=concat
  delay_sync_{1..2,4..5} (4 alike) : xbsIndex_r4/Delay  en=off  latency=1  dbl_ovrd=off  reg_retiming=off  block_type=delay
  delay_sync_3 : xbsIndex_r4/Delay  en=off  latency=35  dbl_ovrd=off  reg_retiming=off  block_type=delay
  coeff_stg1 : Outport
  coeff_stg2 : Outport  Port=2
  coeff_stg3 : Outport  Port=3
  sync_out : Outport  Port=4
  wires:
  sync/1 -> delay_sync_1/1, bulk_delay_1_1/4(in4), bulk_delay_1_1/3(in3), bulk_delay_1_1/2(in2), bulk_delay_1_1/1(in1)
  bulk_delay_1_2/1(out1) -> bulk_delay_2_1/1(in1), coeff_gen_stage_1_group_1/1(sync)
  bulk_delay_1_2/2(out2) -> bulk_delay_2_1/2(in2), coeff_gen_stage_1_group_2/1(sync)
  bulk_delay_1_2/3(out3) -> bulk_delay_2_1/3(in3), coeff_gen_stage_1_group_3/1(sync)
  bulk_delay_1_2/4(out4) -> bulk_delay_2_1/4(in4), coeff_gen_stage_1_group_4/1(sync)
  bulk_delay_2_2/1(out1) -> bulk_delay_3_1/1(in1), coeff_gen_stage_2_group_1/1(sync)
  bulk_delay_2_2/2(out2) -> bulk_delay_3_1/2(in2), coeff_gen_stage_2_group_2/1(sync)
  bulk_delay_2_2/3(out3) -> bulk_delay_3_1/3(in3), coeff_gen_stage_2_group_3/1(sync)
  bulk_delay_2_2/4(out4) -> bulk_delay_3_1/4(in4), coeff_gen_stage_2_group_4/1(sync)
  delay_sync_5/1 -> sync_out/1
  delay_sync_4/1 -> delay_sync_5/1
  delay_sync_3/1 -> delay_sync_4/1
  delay_sync_2/1 -> delay_sync_3/1
  delay_sync_1/1 -> delay_sync_2/1
  concat_stage_3/1 -> coeff_stg3/1
  coeff_gen_stage_3_group_4/1(coeff) -> concat_stage_3/4
  coeff_gen_stage_3_group_3/1(coeff) -> concat_stage_3/3
  coeff_gen_stage_3_group_2/1(coeff) -> concat_stage_3/2
  coeff_gen_stage_3_group_1/1(coeff) -> concat_stage_3/1
  bulk_delay_3_2/4(out4) -> coeff_gen_stage_3_group_4/1(sync)
  bulk_delay_3_2/3(out3) -> coeff_gen_stage_3_group_3/1(sync)
  bulk_delay_3_2/2(out2) -> coeff_gen_stage_3_group_2/1(sync)
  bulk_delay_3_2/1(out1) -> coeff_gen_stage_3_group_1/1(sync)
  bulk_delay_3_1/4(out4) -> bulk_delay_3_2/4(in4)
  bulk_delay_3_1/3(out3) -> bulk_delay_3_2/3(in3)
  bulk_delay_3_1/2(out2) -> bulk_delay_3_2/2(in2)
  bulk_delay_3_1/1(out1) -> bulk_delay_3_2/1(in1)
  concat_stage_2/1 -> coeff_stg2/1
  coeff_gen_stage_2_group_4/1(coeff) -> concat_stage_2/4
  coeff_gen_stage_2_group_3/1(coeff) -> concat_stage_2/3
  coeff_gen_stage_2_group_2/1(coeff) -> concat_stage_2/2
  coeff_gen_stage_2_group_1/1(coeff) -> concat_stage_2/1
  bulk_delay_2_1/4(out4) -> bulk_delay_2_2/4(in4)
  bulk_delay_2_1/3(out3) -> bulk_delay_2_2/3(in3)
  bulk_delay_2_1/2(out2) -> bulk_delay_2_2/2(in2)
  bulk_delay_2_1/1(out1) -> bulk_delay_2_2/1(in1)
  concat_stage_1/1 -> coeff_stg1/1
  coeff_gen_stage_1_group_4/1(coeff) -> concat_stage_1/4
  coeff_gen_stage_1_group_3/1(coeff) -> concat_stage_1/3
  coeff_gen_stage_1_group_2/1(coeff) -> concat_stage_1/2
  coeff_gen_stage_1_group_1/1(coeff) -> concat_stage_1/1
  bulk_delay_1_1/4(out4) -> bulk_delay_1_2/4(in4)
  bulk_delay_1_1/3(out3) -> bulk_delay_1_2/3(in3)
  bulk_delay_1_1/2(out2) -> bulk_delay_1_2/2(in2)
  bulk_delay_1_1/1(out1) -> bulk_delay_1_2/1(in1)

== system monroe_library/FFT_direct/stage_1 ==
  in0_A : Inport
  in0_B : Inport  Port=2
  in1_A : Inport  Port=3
  in1_B : Inport  Port=4
  in2_A : Inport  Port=5
  in2_B : Inport  Port=6
  in3_A : Inport  Port=7
  in3_B : Inport  Port=8
  coeff_arr : Inport  Port=9
  const_sync : xbsIndex_r4/Constant  arith_type=Boolean  const=0  n_bits=16  bin_pt=14  explicit_period=on  period=1  equ=P=C  opselect=C  inp2=PCIN>>17  opr=+  inp1=P  carry=CIN  dbl_ovrd=off  block_type=constant
  twiddle_1x{0..3} (4 alike) : monroe_library/twiddle_cheap  SystemSampleTime=-1  a_n_bits=18  a_bin_pt=17  b_n_bits=18  b_bin_pt=17  w_n_bits=18  w_bin_pt=17  a_delay=0  apbw_delay=0  out_n_bits=18  downshift_at_end=1
  uncram_coeff : Subsystem
  ApBW_0 : Outport
  AmBW_0 : Outport  Port=2
  ApBW_1 : Outport  Port=3
  AmBW_1 : Outport  Port=4
  ApBW_2 : Outport  Port=5
  AmBW_2 : Outport  Port=6
  ApBW_3 : Outport  Port=7
  AmBW_3 : Outport  Port=8
  wires:
  const_sync/1 -> twiddle_1x3/4, twiddle_1x2/4, twiddle_1x1/4, twiddle_1x0/4
  twiddle_1x3/2 -> AmBW_3/1
  twiddle_1x3/1 -> ApBW_3/1
  uncram_coeff/4(out3) -> twiddle_1x3/3
  in3_B/1 -> twiddle_1x3/2
  in3_A/1 -> twiddle_1x3/1
  twiddle_1x2/2 -> AmBW_2/1
  twiddle_1x2/1 -> ApBW_2/1
  uncram_coeff/3(out2) -> twiddle_1x2/3
  in2_B/1 -> twiddle_1x2/2
  in2_A/1 -> twiddle_1x2/1
  twiddle_1x1/2 -> AmBW_1/1
  twiddle_1x1/1 -> ApBW_1/1
  uncram_coeff/2(out1) -> twiddle_1x1/3
  in1_B/1 -> twiddle_1x1/2
  in1_A/1 -> twiddle_1x1/1
  twiddle_1x0/2 -> AmBW_0/1
  twiddle_1x0/1 -> ApBW_0/1
  uncram_coeff/1(out0) -> twiddle_1x0/3
  in0_B/1 -> twiddle_1x0/2
  in0_A/1 -> twiddle_1x0/1
  coeff_arr/1 -> uncram_coeff/1(in)

== system monroe_library/FFT_direct/stage_2 ==
  in0_A : Inport
  in0_B : Inport  Port=2
  in1_A : Inport  Port=3
  in1_B : Inport  Port=4
  in2_A : Inport  Port=5
  in2_B : Inport  Port=6
  in3_A : Inport  Port=7
  in3_B : Inport  Port=8
  coeff_arr : Inport  Port=9
  const_sync : xbsIndex_r4/Constant  arith_type=Boolean  const=0  n_bits=16  bin_pt=14  explicit_period=on  period=1  equ=P=C  opselect=C  inp2=PCIN>>17  opr=+  inp1=P  carry=CIN  dbl_ovrd=off  block_type=constant
  twiddle_2x{0..3} (4 alike) : monroe_library/twiddle_cheap  SystemSampleTime=-1  a_n_bits=18  a_bin_pt=17  b_n_bits=18  b_bin_pt=17  w_n_bits=18  w_bin_pt=17  a_delay=0  apbw_delay=0  out_n_bits=18  downshift_at_end=1
  uncram_coeff : Subsystem
  ApBW_0 : Outport
  AmBW_0 : Outport  Port=2
  ApBW_1 : Outport  Port=3
  AmBW_1 : Outport  Port=4
  ApBW_2 : Outport  Port=5
  AmBW_2 : Outport  Port=6
  ApBW_3 : Outport  Port=7
  AmBW_3 : Outport  Port=8
  wires:
  const_sync/1 -> twiddle_2x3/4, twiddle_2x2/4, twiddle_2x1/4, twiddle_2x0/4
  twiddle_2x3/2 -> AmBW_3/1
  twiddle_2x3/1 -> ApBW_3/1
  uncram_coeff/4(out3) -> twiddle_2x3/3
  in3_B/1 -> twiddle_2x3/2
  in3_A/1 -> twiddle_2x3/1
  twiddle_2x2/2 -> AmBW_2/1
  twiddle_2x2/1 -> ApBW_2/1
  uncram_coeff/3(out2) -> twiddle_2x2/3
  in2_B/1 -> twiddle_2x2/2
  in2_A/1 -> twiddle_2x2/1
  twiddle_2x1/2 -> AmBW_1/1
  twiddle_2x1/1 -> ApBW_1/1
  uncram_coeff/2(out1) -> twiddle_2x1/3
  in1_B/1 -> twiddle_2x1/2
  in1_A/1 -> twiddle_2x1/1
  twiddle_2x0/2 -> AmBW_0/1
  twiddle_2x0/1 -> ApBW_0/1
  uncram_coeff/1(out0) -> twiddle_2x0/3
  in0_B/1 -> twiddle_2x0/2
  in0_A/1 -> twiddle_2x0/1
  coeff_arr/1 -> uncram_coeff/1(in)

== system monroe_library/FFT_direct/stage_3 ==
  in0_A : Inport
  in0_B : Inport  Port=2
  in1_A : Inport  Port=3
  in1_B : Inport  Port=4
  in2_A : Inport  Port=5
  in2_B : Inport  Port=6
  in3_A : Inport  Port=7
  in3_B : Inport  Port=8
  coeff_arr : Inport  Port=9
  const_sync : xbsIndex_r4/Constant  arith_type=Boolean  const=0  n_bits=16  bin_pt=14  explicit_period=on  period=1  equ=P=C  opselect=C  inp2=PCIN>>17  opr=+  inp1=P  carry=CIN  dbl_ovrd=off  block_type=constant
  twiddle_3x{0..3} (4 alike) : monroe_library/twiddle_cheap  SystemSampleTime=-1  a_n_bits=18  a_bin_pt=17  b_n_bits=18  b_bin_pt=17  w_n_bits=18  w_bin_pt=17  a_delay=0  apbw_delay=0  out_n_bits=18  downshift_at_end=1
  uncram_coeff : Subsystem
  ApBW_0 : Outport
  AmBW_0 : Outport  Port=2
  ApBW_1 : Outport  Port=3
  AmBW_1 : Outport  Port=4
  ApBW_2 : Outport  Port=5
  AmBW_2 : Outport  Port=6
  ApBW_3 : Outport  Port=7
  AmBW_3 : Outport  Port=8
  wires:
  const_sync/1 -> twiddle_3x3/4, twiddle_3x2/4, twiddle_3x1/4, twiddle_3x0/4
  twiddle_3x3/2 -> AmBW_3/1
  twiddle_3x3/1 -> ApBW_3/1
  uncram_coeff/4(out3) -> twiddle_3x3/3
  in3_B/1 -> twiddle_3x3/2
  in3_A/1 -> twiddle_3x3/1
  twiddle_3x2/2 -> AmBW_2/1
  twiddle_3x2/1 -> ApBW_2/1
  uncram_coeff/3(out2) -> twiddle_3x2/3
  in2_B/1 -> twiddle_3x2/2
  in2_A/1 -> twiddle_3x2/1
  twiddle_3x1/2 -> AmBW_1/1
  twiddle_3x1/1 -> ApBW_1/1
  uncram_coeff/2(out1) -> twiddle_3x1/3
  in1_B/1 -> twiddle_3x1/2
  in1_A/1 -> twiddle_3x1/1
  twiddle_3x0/2 -> AmBW_0/1
  twiddle_3x0/1 -> ApBW_0/1
  uncram_coeff/1(out0) -> twiddle_3x0/3
  in0_B/1 -> twiddle_3x0/2
  in0_A/1 -> twiddle_3x0/1
  coeff_arr/1 -> uncram_coeff/1(in)

== system monroe_library/biplex_4x_unscr/dual_bit_reverse ==
  sync : Inport
  din0 : Inport  Port=2
  din1 : Inport  Port=3
  Concat1 : xbsIndex_r4/Concat  num_inputs=2  dbl_ovrd=off  block_type=concat
  Concat2 : xbsIndex_r4/Concat  num_inputs=2  dbl_ovrd=off  block_type=concat
  Constant : xbsIndex_r4/Constant  arith_type=Boolean  const=1  n_bits=1  bin_pt=0  explicit_period=on  period=1  equ=P=C  opselect=C  inp2=PCIN>>17  opr=+  inp1=P  carry=CIN  dbl_ovrd=off  block_type=constant
  Constant1 : xbsIndex_r4/Constant  arith_type=Boolean  const=0  n_bits=1  bin_pt=0  explicit_period=on  period=1  equ=P=C  opselect=C  inp2=PCIN>>17  opr=+  inp1=P  carry=CIN  dbl_ovrd=off  block_type=constant
  Constant5 : xbsIndex_r4/Constant  arith_type=Boolean  const=1  n_bits=1  bin_pt=0  explicit_period=on  period=1  equ=P=C  opselect=C  inp2=PCIN>>17  opr=+  inp1=P  carry=CIN  dbl_ovrd=off  block_type=constant
  Counter : xbsIndex_r4/Counter  cnt_type=Free Running  cnt_to=1023  operation=Up  start_count=0  cnt_by_val=1  arith_type=Unsigned  n_bits=9  bin_pt=0  load_pin=off  rst=on  en=off  explicit_period=on  period=1  dbl_ovrd=off  use_behavioral_HDL=off  implementation=Fabric  use_rpm=off  block_type=counter
  Counter1 : xbsIndex_r4/Counter  cnt_type=Free Running  cnt_to=1023  operation=Down  start_count=511  cnt_by_val=1  arith_type=Unsigned  n_bits=9  bin_pt=0  load_pin=off  rst=on  en=off  explicit_period=on  period=1  dbl_ovrd=off  use_behavioral_HDL=off  implementation=Fabric  use_rpm=off  block_type=counter
  Dual Port RAM : xbsIndex_r4/Dual Port RAM  depth=512  initVector=sin(pi*(0:15)/16)  distributed_mem=Block RAM  init_a=0  init_b=0  rst_a=off  rst_b=off  en_a=off  en_b=off  latency=3  write_mode_A=Read Before Write  write_mode_B=Read Before Write  dbl_ovrd=off  optimize=Area  use_rpm=on  block_type=dpram
  Inverter : xbsIndex_r4/Inverter  en=off  latency=0  dbl_ovrd=off  block_type=inv
  Mux : xbsIndex_r4/Mux  inputs=2  en=off  latency=0  precision=Full  arith_type=Unsigned  n_bits=16  bin_pt=14  quantization=Truncate  overflow=Wrap  dbl_ovrd=off  block_type=mux
  Mux1 : xbsIndex_r4/Mux  inputs=2  en=off  latency=0  precision=Full  arith_type=Unsigned  n_bits=16  bin_pt=14  quantization=Truncate  overflow=Wrap  dbl_ovrd=off  block_type=mux
  Slice1 : xbsIndex_r4/Slice  nbits=1  boolean_output=off  mode=Upper Bit Location + Width  bit1=0  base1=MSB of Input  bit0=0  base0=LSB of Input  dbl_ovrd=off  block_type=slice
  Slice2 : xbsIndex_r4/Slice  nbits=8  boolean_output=off  mode=Lower Bit Location + Width  bit1=0  base1=MSB of Input  bit0=0  base0=LSB of Input  dbl_ovrd=off  block_type=slice
  Slice3 : xbsIndex_r4/Slice  nbits=1  boolean_output=off  mode=Upper Bit Location + Width  bit1=0  base1=MSB of Input  bit0=0  base0=LSB of Input  dbl_ovrd=off  block_type=slice
  Slice4 : xbsIndex_r4/Slice  nbits=8  boolean_output=off  mode=Lower Bit Location + Width  bit1=0  base1=MSB of Input  bit0=0  base0=LSB of Input  dbl_ovrd=off  block_type=slice
  bit_reverse_1 : Subsystem
  bit_reverse_2 : Subsystem
  delay_din0 : xbsIndex_r4/Delay  en=off  latency=1  dbl_ovrd=off  reg_retiming=off  block_type=delay
  delay_din1 : xbsIndex_r4/Delay  en=off  latency=1  dbl_ovrd=off  reg_retiming=off  block_type=delay
  post_sync_delay : xbsIndex_r4/Delay  en=off  latency=3  dbl_ovrd=off  reg_retiming=off  block_type=delay
  post_sync_delay1 : xbsIndex_r4/Delay  en=off  latency=1  dbl_ovrd=off  reg_retiming=off  block_type=delay
  sync_delay_fast : monroe_library/sync_delay_fast  SystemSampleTime=-1  delay_len=256
  sync_out : Outport
  dout0 : Outport  Port=2
  dout1 : Outport  Port=3
  wires:
  Constant/1 -> Dual Port RAM/6, Dual Port RAM/3
  Counter/1 -> Slice2/1, Slice1/1
  Slice1/1 -> Mux1/1, Mux/1
  Slice2/1 -> bit_reverse_1/1(in), Mux1/2, Mux/2
  Counter1/1 -> Slice4/1, Slice3/1
  post_sync_delay1/1 -> sync_delay_fast/1, Counter1/1, Counter/1
  bit_reverse_2/1(out) -> Mux1/3
  Slice4/1 -> bit_reverse_2/1(in)  "xlsub3_Slice4_out1"
  bit_reverse_1/1(out) -> Mux/3
  sync_delay_fast/1 -> post_sync_delay/1
  sync/1 -> post_sync_delay1/1
  post_sync_delay/1 -> sync_out/1
  delay_din1/1 -> Dual Port RAM/5
  din1/1 -> delay_din1/1
  delay_din0/1 -> Dual Port RAM/2
  din0/1 -> delay_din0/1
  Slice3/1 -> Inverter/1
  Mux1/1 -> Concat1/2
  Mux/1 -> Concat2/2
  Dual Port RAM/2 -> dout1/1
  Dual Port RAM/1 -> dout0/1
  Concat1/1 -> Dual Port RAM/4
  Concat2/1 -> Dual Port RAM/1
  Constant5/1 -> Concat2/1
  Constant1/1 -> Concat1/1
